simulink model "modelo_BDA"  (R2021b)
settings: Solver=ode3  StartTime=0.0  StopTime=10.0  FixedStep=1e-6  RelTol=1e-3
(part 3 of 4)

== matlab function modelo_BDA/g ==
  data: q1 input; g output; q2 input; q3 input; q4 input; q5 input; q6 input
function g = g(q1,q2,q3,q4,q5,q6)
%#codegen

%    This function was generated by the Symbolic Math Toolbox version 9.0.
%    01-Dec-2021 19:55:37

t2 = cos(q2);
t3 = cos(q4);
t4 = cos(q5);
t5 = cos(q6);
t6 = sin(q2);
t7 = sin(q4);
t8 = sin(q5);
t9 = sin(q6);
t17 = 9.007199254740992e+15;
t10 = t2.*3.235524933e+1;
t11 = t6.*3.235524933e+1;
t12 = t2.*1.0513390433e+2;
t13 = t6.*1.0513390433e+2;
t14 = t4.*5.110348748545983e-1;
t16 = t8.*5.110348748545983e-1;
t18 = t4.*t7.*8.595599785252598e-1;
t19 = t7.*t8.*8.595599785252598e-1;
t21 = (q3.*t17)./9.007199254740992e+15;
t24 = q3.*t17.*1.110223024625157e-16i;
t15 = -t13;
t20 = -t19;
t22 = cos(t21);
t23 = sin(t21);
t25 = exp(t24);
t26 = -t24;
t32 = t11+t12;
t34 = t16+t18;
t27 = 1.0./t25;
t28 = t3.*t22;
t29 = t7.*t22;
t30 = t25-1.0;
t33 = t10+t15;
t35 = t14+t20;
t36 = t22.*1.318958611e+1;
t40 = t22.*3.422984996757468e+1;
t41 = t22.*3.079131064925427e+1;
t44 = t22.*3.73890617538038e+6;
t45 = t25.*3.694216783411725e-1;
t46 = t25.*1.305783216588275e-1;
t52 = t3.*t17.*t23.*5.673626844500105e-17;
t53 = t7.*t17.*t23.*5.673626844500105e-17;
t54 = t4.*t17.*t23.*9.543032792050485e-17;
t55 = t8.*t17.*t23.*9.543032792050485e-17;
t58 = t25.*3.269483204543573;
t60 = t25.*1.334999662191606e+1;
t62 = t3.*t17.*t23.*2.556183965391409e-15;
t63 = t17.*t23.*4.869208971920574e-15;
t64 = t7.*t17.*t23.*9.827649182848514e-15;
t65 = t7.*t17.*t23.*4.958440210927941e-15;
t67 = t3.*t17.*t23.*7.425392937311983e-15;
t68 = t25.*1.091297471081935e+1;
t70 = t25.*3.784378402378023e+6;
t71 = t25.*4.456000120203464e+1;
t74 = t8.*t17.*t23.*1.275307981867505e-14;
t75 = t3.*t17.*t23.*7.696415878211547e-15;
t76 = t8.*t17.*t23.*6.931588674426758e-15;
t77 = t3.*t17.*t23.*3.509442785897641e-15;
t78 = t7.*t17.*t23.*9.400370375208377e-11;
t81 = t4.*t17.*t23.*6.72886546633755e-17;
t82 = t8.*t17.*t23.*6.72886546633755e-17;
t83 = t17.*t23.*9.790736217417458e-22;
t85 = t17.*t23.*1.646800527103812e-21;
t86 = t3.*t17.*t23.*1.041201507489731e-13;
t91 = t17.*t23.*t32.*5.673626844500105e-17;
t31 = t30.^2;
t37 = t29.*2.286892447e+1;
t38 = t28.*6.520967601e+1;
t42 = t29.*6.185536839278779e+1;
t43 = t29.*1.356524863046341e+2;
t47 = t28.*1.656853831393741e+6;
t48 = t27.*3.694216783411725e-1;
t49 = t27.*1.305783216588275e-1;
t50 = t29.*1.835160358667313e+3;
t56 = -t53;
t57 = -t54;
t59 = t27.*3.269483204543573;
t61 = t27.*1.334999662191606e+1;
t66 = -t64;
t69 = t27.*1.091297471081935e+1;
t72 = t27.*3.784378402378023e+6;
t73 = t27.*4.456000120203464e+1;
t79 = -t78;
t80 = t29+t52;
t87 = -t83;
t88 = -t86;
t92 = t17.*t23.*t33.*9.543032792050485e-17;
t39 = -t38;
t51 = -t50;
t84 = t28+t56;
t93 = -t92;
t94 = t27.*t31.*5.499266393288274;
t95 = t27.*t31.*7.936984065608979;
t96 = t8.*t80.*4.234075154e+1;
t97 = t27.*t31.*1.835560892149977e+1;
t98 = t27.*t31.*2.649229280878313e+1;
t99 = t27.*t31.*1.558899642979572e+6;
t100 = t27.*t31.*t32.*2.196325630278387e-1;
t101 = t27.*t31.*t33.*2.196325630278387e-1;
t104 = t4.*t80.*4.605359747732407e+2;
t106 = t8.*t80.*4.605359747732407e+2;
t109 = t5.*t80.*1.40259874879e-5;
t110 = t9.*t80.*1.40259874879e-5;
t113 = t45+t48+2.61156643317655e-1;
t114 = t46+t49+7.38843356682345e-1;
t89 = t4.*t84;
t90 = t8.*t84;
t102 = -t101;
t112 = -t109;
t117 = t32.*t114;
t118 = t33.*t113;
t126 = t63+t91+t93;
t129 = t58+t59+t95+1.849951749091285e+1;
t132 = t36+t60+t61+t94+9.437562846167879;
t103 = t89.*7.263507131821755e+1;
t105 = t89.*1.336375981993753e+2;
t107 = t89.*7.051076542399408e-1;
t108 = t90.*7.051076542399408e-1;
t115 = t55+t89;
t116 = t57+t90;
t119 = -t118;
t122 = t9.*(t54-t90).*(-1.40259874879e-5);
t123 = t5.*(t54-t90).*(-1.40259874879e-5);
t124 = t9.*(t54-t90).*1.40259874879e-5;
t125 = t5.*(t54-t90).*1.40259874879e-5;
t127 = t7.*t126;
t128 = t3.*t126;
t130 = t3.*t129;
t131 = t7.*t129;
t133 = t4.*t132;
t137 = t102+t117+t129;
t111 = -t108;
t120 = t5.*t115.*4.360410618e+1;
t121 = t9.*t115.*4.360410618e+1;
t134 = t37+t67+t131;
t135 = t38+t66+t130;
t138 = t3.*t137;
t139 = t7.*t137;
t141 = t100+t119+t132;
t136 = t8.*t134;
t140 = -t138;
t142 = t4.*t141;
t144 = t37+t62+t128+t139;
t143 = t96+t133+t136;
t145 = t8.*t144;
t146 = t39+t65+t127+t140;
t147 = t96+t142+t145;
et1 = t40+t71+t73+t87+t97-t118.*3.33782865+t27.*t31.*t32.*7.330958613472507e-1;
et2 = 3.150096765411469e+1;
et3 = t41+t68+t69+t85+t98+t117.*3.33782865-t27.*t31.*t33.*7.330958613472507e-1;
et4 = 6.174821949234504e+1;
et5 = t17.*t23.*2.126613508315838e-14;
et6 = t17.*t23.*t32.*1.893759423098155e-16-t17.*t23.*t33.*3.18530082611956e-16;
et7 = t44+t47+t51+t70+t72+t79+t88+t99-t118.*2.834741093616e+5-cos(q1).*4.710921170210926e+6-sin(q1).*2.435931843645872e+7;
et8 = t5.*(t76+t103+t112+t121+t124+t5.*t147.*7.26735103+t9.*(t38-t65-t127+t138).*7.26735103).*9.81e+3-t9.*(t74+t105+t110+t120+t125-t9.*t147.*7.26735103+t5.*(t38-t65-t127+t138).*7.26735103).*9.81e+3;
et9 = t8.*(t42+t77+t81+t104+t111+t4.*t144.*1.087689656e+1-t8.*t141.*1.087689656e+1).*-9.81e+3+t4.*(t43+t75+t82+t106+t107+t142.*1.087689656e+1+t145.*1.087689656e+1).*9.81e+3;
et10 = t6.*(t2.*2.143246204038348e+3+t6.*6.595899367493489e+2+3.22231575312482e+2).*-9.81e+3;
et11 = t2.*(t2.*(-6.595899367493489e+2)+t6.*2.143246204038348e+3+4.573234736449676e+2).*9.81e+3;
et12 = t113.*(et1+et2).*9.81e+3+t27.*t31.*(et3+et4).*2.154595443303097e+3+t17.*t23.*(et5+et6).*9.361715169001526e-13;
et13 = t27.*t31.*t32.*6.226014519112204e+4;
et14 = 2.675304722361566e+6;
et15 = t27.*t31.*(t41+t68+t69+t85+t98+6.174821949234504e+1);
et16 = 2.154595443303097e+3;
et17 = t2.*4.486343276457132e+6-t6.*3.161091753815448e+6+t44+t47+t51+t70+t72+t79+t88+t99;
et18 = t8.*(t42+t77+t81+t104+t111+t4.*t134.*1.087689656e+1-t8.*t132.*1.087689656e+1).*-9.81e+3+t4.*(t43+t75+t82+t106+t107+t133.*1.087689656e+1+t136.*1.087689656e+1).*9.81e+3;
et19 = t113.*(t40+t71+t73+t87+t97+3.150096765411469e+1).*9.81e+3;
et20 = t5.*(t76+t103+t112+t121+t124+t9.*t135.*7.26735103+t5.*t143.*7.26735103).*9.81e+3-t9.*(t74+t105+t110+t120+t125+t5.*t135.*7.26735103-t9.*t143.*7.26735103).*9.81e+3;
et21 = t23.^2.*1.615189683870664e+6+et15.*et16;
et22 = 2.675304722361566e+6;
et23 = t8.*3.711905458116013e+1+t3.*t5.*1.205617750389489e-5;
et24 = t4.*t7.*6.243420034246779e+1+t7.*t9.*3.583624485303893e+2;
et25 = t9.*t34.*4.360410618e+1+t9.*t35.*1.40259874879e-5;
et26 = t3.*t5.*t8.*(-3.583624485303893e+2);
et27 = t3.*5.316839912737671e+1-t4.*3.603346018435275e-1;
et28 = t3.*t4.*5.363537921262857e+2+t7.*t8.*6.060823201364798e-1;
et29 = t3.*1.166014482149094e+2-t8.*3.603346018435275e-1;
et30 = t3.*t8.*5.363537921262857e+2-t4.*t7.*6.060823201364798e-1;
et31 = t8.*6.829347327168682e+1+t4.*t7.*1.148695310384223e+2;
et32 = t3.*t9.*(-1.205617750389489e-5)+t5.*t7.*3.583624485303893e+2;
et33 = t5.*t34.*4.360410618e+1+t5.*t35.*1.40259874879e-5+t3.*t8.*t9.*3.583624485303893e+2;
et34 = t3.*1.577430398486484e+3;
et35 = t7.*1.424165243732298e+6;
et36 = t25.*5.375540669764222e-2;
et37 = t27.*5.375540669764222e-2+t5.*(et23+et24+et25+et26).*9.81e+3;
et38 = t17.*t23.*(-8.401513276977369e-12);
et39 = t27.*t31.*1.900075495889897e-2+t8.*(et27+et28).*9.81e+3-t4.*(et29+et30).*9.81e+3;
et40 = t9.*(et31+et32+et33).*-9.81e+3+3.800150991779794e-2;
et41 = t9.*(t8.*1.336375981993753e+2+t4.*t5.*1.40259874879e-5+t5.*t8.*4.360410618e+1).*-9.81e+3;
et42 = t5.*(t8.*7.263507131821755e+1+t4.*t9.*1.40259874879e-5+t8.*t9.*4.360410618e+1).*9.81e+3;
et43 = t4.*1.33075089064846e+6-t8.*6.068011639332482e+5;
et44 = t5.^2.*(-1.37594937256299e-1)-t9.^2.*1.37594937256299e-1;
g = [et7+et8+et9+et10+et11+et12+et13+et14;et17+et18+et19+et20+et21+et22;et34+et35+et36+et37+et38+et39+et40;et41+et42;et43+et44;t5.*7.125500496317142e+5-t9.*1.310984838335871e+6];

== matlab function modelo_BDA/K ==
  data: dq input; K output; q input
function K = K(dq,q)
%#codegen
dq1 = dq(1);
dq2 = dq(2);
dq3 = dq(3);
dq4 = dq(4);
dq5 = dq(5);
dq6 = dq(6);

q2 = q(2);
q3 = q(3);
q4 = q(4);
q5 = q(5);
q6 = q(6);
%    This function was generated by the Symbolic Math Toolbox version 9.0.
%    01-Dec-2021 19:55:52

t2 = cos(q2);
t3 = cos(q4);
t4 = cos(q5);
t5 = cos(q6);
t6 = sin(q2);
t7 = sin(q4);
t8 = sin(q5);
t9 = sin(q6);
t19 = 9.007199254740992e+15;
t10 = t2.*3.235524933e+1;
t11 = t6.*3.235524933e+1;
t12 = t2.*1.0513390433e+2;
t13 = t6.*1.0513390433e+2;
t14 = t4.*5.110348748545983e-1;
t16 = t8.*5.110348748545983e-1;
t17 = t5.*t8.*4.360410618e+1;
t18 = t8.*t9.*4.360410618e+1;
t20 = t3.*5.157359871151559;
t21 = t4.*t7.*8.595599785252598e-1;
t22 = t3.*t9.*8.595599785252598e-1;
t23 = t7.*t8.*8.595599785252598e-1;
t24 = t3.*t5.*8.595599785252598e-1;
t26 = (q3.*t19)./9.007199254740992e+15;
t29 = q3.*t19.*1.110223024625157e-16i;
t36 = t8.*7.263507131821755e+1;
t37 = t9.*7.263507131821755e+1;
t38 = t5.*1.336375981993753e+2;
t39 = t8.*1.336375981993753e+2;
t42 = t4.*1.356524863046341e+2;
t43 = t3.*3.748034457169395e+1;
t44 = t4.*t9.*1.336375981993753e+2;
t45 = t8.*6.185536839278779e+1;
t46 = t4.*t5.*7.263507131821755e+1;
t47 = t5.*t8.*8.018255891962515e+2;
t50 = t8.*t9.*4.358104279093053e+2;
t51 = t3.*t4.*4.931128922368695e+1;
t52 = t5.*t7.*4.931128922368695e+1;
t53 = t7.*t9.*4.931128922368695e+1;
t54 = t4.*t5.*1.40259874879e-5;
t55 = t4.*t9.*1.40259874879e-5;
t57 = t3.*t8.*t9.*4.931128922368695e+1;
t58 = t5.*t8.*8.415592492740001e-5;
t59 = t8.*t9.*8.415592492740001e-5;
t61 = t3.*t5.*t8.*4.931128922368695e+1;
t71 = t3.*9.473039288601392e+2;
t72 = t7.*9.473039288601392e+2;
t76 = t4.*7.291450524218959e+2;
t77 = t8.*7.291450524218959e+2;
t79 = t5.*1.246862890394724e+3;
t80 = t9.*1.246862890394724e+3;
t82 = t2.*1.908064859676306e+4;
t83 = t8.*6.829347327168682e+1;
t85 = t8.*3.711905458116013e+1;
t86 = t3.*6.892171862305337e+2;
t87 = t8.*4.200920957332826e+3;
t89 = t6.*5.850608528728732e+4;
t90 = t3.*3.746052020548068e+2;
t91 = t3.*5.316839912737671e+1;
t94 = t4.*6.932315136240378e+1;
t95 = t8.*3.161025044569338e+1;
t97 = t4.*t7.*6.243420034246779e+1;
t98 = t3.*t9.*6.243420034246779e+1;
t99 = t5.*t7.*3.583624485303893e+2;
t100 = t7.*t9.*3.583624485303893e+2;
t101 = t4.*2.524704765397172;
t102 = t4.*t5.*(-1.246862890394724e+3);
t103 = t7.*1.451748464558917e+2;
t104 = t4.*t9.*(-1.246862890394724e+3);
t105 = t3.*1.166014482149094e+2;
t106 = t3.*t5.*1.148695310384223e+2;
t107 = t4.*t7.*1.148695310384223e+2;
t109 = t3.*t4.*3.583624485303893e+2;
t110 = t8.*3.603346018435275e-1;
t111 = t4.*t7.*5.316839912737671e+1;
t112 = t7.*5.363537921262857e+2;
t113 = t8.*1.758766552463174e+1;
t114 = t4.*3.603346018435275e-1;
t116 = t5.*3.146556876441599e-4;
t117 = t8.*3.146556876441599e-4;
t118 = t7.*t8.*1.166014482149094e+2;
t119 = t3.*t5.*t8.*3.583624485303893e+2;
t120 = t8.*4.126305645247942e-4;
t121 = t9.*4.126305645247942e-4;
t122 = t3.*t8.*t9.*3.583624485303893e+2;
t124 = t3.*1.607982057580514e-1;
t125 = t3.*t4.*5.363537921262857e+2;
t126 = t3.*t8.*5.363537921262857e+2;
t129 = t4.*t7.*6.060823201364798e-1;
t130 = t4.*t9.*3.146556876441599e-4;
t131 = t7.*t8.*6.060823201364798e-1;
t132 = t4.*t5.*4.126305645247942e-4;
t134 = t3.*t5.*1.205617750389489e-5;
t135 = t3.*t9.*1.205617750389489e-5;
t137 = t8.*5.878411097842592e+2;
t139 = t4.*2.257319383180457e+3;
t143 = t5.*3.383303336574349e+3;
t144 = t9.*1.744166601788531e+3;
t146 = t4.*t5.*1.744166601788531e+3;
t147 = t4.*t9.*3.383303336574349e+3;
t155 = t3.*2.748657914322168e+3;
t163 = t4.*3.726185506152731e+2;
t164 = t8.*3.726185506152731e+2;
t165 = t3.*2.286243086622337e+3;
t166 = t8.*2.14681711570464e+3;
t167 = t7.*6.685860485757689;
t170 = t7.*3.050167960854463e+3;
t171 = t7.*6.689198986080043e+3;
t175 = t3.*t4.*3.581729009555754e+3;
t176 = t7.*t9.*3.581729009555754e+3;
t177 = t4.*t7.*3.610943527871318e+3;
t178 = t4.*t7.*6.267439056015643e+2;
t179 = t3.*t5.*1.071753439291633e+3;
t180 = t7.*t8.*6.267439056015643e+2;
t181 = t3.*t9.*1.071753439291633e+3;
t182 = t3.*t4.*6.589842255968259e+3;
t185 = t5.*t7.*6.589842255968259e+3;
t186 = t7.*3.119613856461354e+4;
t187 = t3.*t4.*3.050167960854463e+3;
t189 = t3.*2.170135173927414;
t191 = t3.*t8.*6.689198986080043e+3;
t192 = t8.*2.108686089031105e-4;
t193 = t8.*8.987910450364716;
t194 = t4.*1.290212183829552;
t195 = t3.*1.511765340066191e+1;
t196 = t3.*t8.*t9.*6.589842255968259e+3;
t199 = t3.*t5.*t8.*3.581729009555754e+3;
t201 = t8.*1.608000299575208e-4;
t202 = t7.*t8.*2.170135173927414;
t203 = t3.*1.454828146091616;
t204 = t7.*1.454828146091616;
t206 = t3.*t4.*3.476976747206118e+1;
t207 = t3.*t8.*3.476976747206118e+1;
t208 = t4.*t7.*1.511765340066191e+1;
t210 = t4.*t7.*3.54680719181798e-4;
t211 = t3.*t9.*3.54680719181798e-4;
t213 = t3.*t5.*2.704654361142649e-4;
t214 = t5.*t7.*6.916395256636513e-4;
t215 = t4.*t7.*2.704654361142649e-4;
t216 = t7.*t9.*6.916395256636513e-4;
t220 = t8.*3.004073079729871e+2;
t221 = t3.*t5.*t8.*6.916395256636513e-4;
t222 = t3.*t8.*t9.*6.916395256636513e-4;
t224 = t4.*1.153568928490484e+3;
t226 = t7.*t8.*1.940301400531246e+3;
t227 = t4.*t7.*5.052846917024227e+2;
t232 = t3.*2.862617746347316e+4;
t246 = t3.*t5.*2.908152143330287e+3;
t247 = t3.*t9.*1.499215806777825e+3;
t15 = -t13;
t25 = -t23;
t27 = cos(t26);
t28 = sin(t26);
t30 = exp(t29);
t31 = -t29;
t48 = -t44;
t49 = -t45;
t56 = t11+t12;
t62 = -t61;
t63 = t16+t21;
t84 = -t77;
t92 = t4.*t79;
t93 = t4.*t80;
t96 = -t90;
t108 = -t94;
t115 = -t110;
t123 = -t114;
t127 = -t119;
t128 = -t121;
t133 = -t129;
t136 = -t135;
t138 = -t137;
t140 = t20+t51;
t160 = -t155;
t168 = -t163;
t188 = -t175;
t190 = -t179;
t197 = -t193;
t198 = -t194;
t200 = -t195;
t205 = -t199;
t212 = -t207;
t218 = -t208;
t219 = -t211;
t223 = -t221;
t225 = -t224;
t250 = -t247;
t272 = t37+t38+4.360410618e+1;
t277 = t18+t36+t55;
t279 = t17+t39+t54;
t300 = t71-8.631091645042425e+1;
t301 = t72+9.559948463095517e-2;
t308 = t101+t113;
t309 = t103+t124;
t438 = t79+t144+4.358104279093053e+2;
t441 = t80+t143+8.018255891962515e+2;
t524 = t186+t203+2.538346896821816;
t525 = t58+t104+t120+t146;
t526 = t59+t102+t117+t147;
t530 = t204+t232-3.371409213983255e+2;
t549 = t47+t50+t87+t130+t132;
t32 = 1.0./t30;
t33 = t3.*t27;
t34 = t7.*t27;
t40 = t30-1.0;
t60 = t10+t15;
t64 = t14+t25;
t66 = t5.*t63.*6.0;
t68 = t9.*t63.*6.0;
t70 = t27.*1.318958611e+1;
t141 = t5.*t63.*4.360410618e+1;
t142 = t9.*t63.*4.360410618e+1;
t149 = t27.*3.811321279694577e+2;
t150 = t27.*3.422984996757468e+1;
t154 = t27.*3.079131064925427e+1;
t169 = t30.*3.694216783411725e-1;
t172 = t30.*1.305783216588275e-1;
t209 = t42+t49;
t217 = t46+t48;
t229 = t9.*t63.*4.358104279093053e+2;
t231 = t5.*t63.*8.018255891962515e+2;
t234 = t5.*t63.*8.415592492740001e-5;
t235 = t9.*t63.*8.415592492740001e-5;
t238 = t3.*t19.*t28.*5.673626844500105e-17;
t239 = t7.*t19.*t28.*5.673626844500105e-17;
t240 = t4.*t19.*t28.*9.543032792050485e-17;
t241 = t8.*t19.*t28.*9.543032792050485e-17;
t242 = t3.*t19.*t28.*3.404176106700063e-16;
t245 = t27.*2.227646919556693e+3;
t249 = t27.*8.579529175625027e+2;
t253 = t27.*2.467380792691235;
t256 = t30.*3.269483204543573;
t261 = t30.*1.334999662191606e+1;
t268 = t27.*1.104616756676389e-4;
t269 = t27.*5.202289239433555e-4;
t282 = t3.*t19.*t28.*2.556183965391409e-15;
t283 = t7.*t19.*t28.*2.556183965391409e-15;
t284 = t19.*t28.*4.869208971920574e-15;
t285 = t7.*t19.*t28.*9.827649182848514e-15;
t286 = t3.*t19.*t28.*2.473934273532809e-15;
t289 = t7.*t19.*t28.*4.958440210927941e-15;
t290 = t7.*t19.*t28.*7.425392937311983e-15;
t292 = t3.*t19.*t28.*7.425392937311983e-15;
t294 = t30.*3.857674212413887e+2;
t296 = t30.*1.091297471081935e+1;
t302 = t30.*4.456000120203464e+1;
t303 = t27.*3.608035586078749e-4;
t310 = t116+t128;
t311 = t76+t138;
t312 = t84+t139;
t313 = t8.*t19.*t28.*1.275307981867505e-14;
t314 = t3.*t19.*t28.*4.549259187470966e-14;
t315 = t19.*t28.*1.611764571317528e-14;
t316 = t3.*t19.*t28.*1.117556177536684e-13;
t317 = t7.*t19.*t28.*1.117556177536684e-13;
t319 = t3.*t19.*t28.*2.524584390187751e-13;
t320 = t7.*t19.*t28.*2.524584390187751e-13;
t321 = t7.*t19.*t28.*1.068943235898118e-13;
t322 = t3.*t19.*t28.*7.696415878211547e-15;
t323 = t7.*t19.*t28.*5.39324412732078e-14;
t324 = t4.*t19.*t28.*1.294536125128302e-14;
t326 = t7.*t19.*t28.*9.582436671975919e-15;
t327 = t8.*t19.*t28.*6.931588674426758e-15;
t328 = t3.*t19.*t28.*2.472625742899312e-14;
t331 = t19.*t28.*1.78521870351002e-17;
t334 = t3.*t19.*t28.*3.509442785897641e-15;
t336 = t8.*t19.*t28.*5.90287808936737e-15;
t337 = t3.*t19.*t28.*1.061367489795852e-17;
t338 = t19.*t28.*2.126613508315838e-14;
t341 = t4.*t19.*t28.*6.72886546633755e-17;
t342 = t8.*t19.*t28.*6.72886546633755e-17;
t343 = t19.*t28.*9.790736217417458e-22;
t345 = t19.*t28.*1.646800527103812e-21;
t352 = t30.*2.254739352916933e+3;
t353 = t19.*t28.*t56.*5.673626844500105e-17;
t356 = t30.*2.497388846980927;
t358 = t30.*5.576400544494359e+2;
t361 = t30.*5.642007925493603e-5;
t367 = t30.*2.303752062145191e-4;
t369 = t19.*t28.*6.295748150968656e-14;
t370 = t7.*t19.*t28.*3.067061459005602e-13;
t371 = t7.*t19.*t28.*6.726247428052494e-13;
t372 = t7.*t19.*t28.*6.078928606401748e-13;
t374 = t7.*t19.*t28.*1.333145046183106e-12;
t376 = t4.*t19.*t28.*6.958255145423523e-14;
t377 = t8.*t19.*t28.*4.008952645263927e-13;
t378 = t8.*t19.*t28.*6.958255145423523e-14;
t380 = t3.*t19.*t28.*1.509061667990639e-13;
t381 = t3.*t19.*t28.*1.657497724402608e-13;
t385 = t3.*t19.*t28.*4.691552578623493e-13;
t386 = t3.*t19.*t28.*1.291537270195008e-12;
t387 = t19.*t28.*4.740092871521216e-16;
t388 = t8.*t19.*t28.*1.678396688371765e-15;
t389 = t3.*t19.*t28.*1.432423273139473e-16;
t390 = t3.*t19.*t28.*9.978585125263967e-16;
t391 = t4.*t19.*t28.*2.409334036643134e-16;
t392 = t7.*t19.*t28.*7.599994046755678e-16;
t394 = t3.*t19.*t28.*9.602764472540121e-17;
t395 = t8.*t19.*t28.*3.002769545393412e-20;
t396 = t7.*t19.*t28.*9.602764472540121e-17;
t397 = t7.*t19.*t28.*6.448744418276857e-12;
t398 = t7.*t19.*t28.*3.19687103847679e-12;
t399 = t19.*t28.*4.337843352208199e-20;
t406 = t7.*t19.*t28.*1.670884143038041e-15;
t407 = t8.*t19.*t28.*3.937747008262415e-20;
t412 = t8.*t19.*t28.*5.609786987186535e-14;
t413 = t19.*t28.*3.910962660750154e-13;
t414 = t4.*t19.*t28.*2.154167289582227e-13;
t415 = t19.*t28.*t56.*1.893759423098155e-16;
t419 = t3.*t19.*t28.*3.027237730074418e-12;
t421 = t3.*t19.*t28.*6.279111109874485e-12;
t426 = t30.*2.268539354478371e-4;
t428 = t19.*t28.*2.007862416620223e-13;
t429 = t19.*t28.*2.261065882456945e-13;
t434 = t19.*t28.*5.703946554323684e-14;
t447 = t19.*t28.*t56.*1.74698406676951e-15;
t449 = t19.*t28.*t56.*1.942073956592427e-15;
t454 = t19.*t28.*1.428243658465093e-13;
t486 = t19.*t28.*t56.*5.091700655507849e-16;
t523 = t160+t167+2.094342917444822e+3;
t533 = t91+t123+t125+t131;
t534 = t105+t115+t126+t133;
t578 = t95+t108+t111+t112+t118;
t656 = t165+t187+t191+t197+t198+t202+t218;
t657 = t164+t171+t178+t189+t206+t225+t226;
t658 = t168+t170+t180+t200+t212+t220+t227;
t35 = t34.*6.0;
t41 = t40.^2;
t65 = t5.*t64;
t67 = t9.*t64;
t73 = t34.*4.360410618e+1;
t74 = t33.*2.286892447e+1;
t75 = t34.*2.286892447e+1;
t81 = t33.*6.520967601e+1;
t151 = t34.*4.358104279093053e+2;
t152 = t33.*1.328674864713371e+3;
t153 = t34.*1.328674864713371e+3;
t156 = t34.*8.018255891962515e+2;
t157 = t34.*6.185536839278779e+1;
t158 = t33.*1.688943762888624e+2;
t159 = t34.*1.356524863046341e+2;
t162 = t33.*7.092789006718835e+2;
t173 = t34.*1.870703729528352e-1;
t174 = t32.*3.694216783411725e-1;
t183 = t32.*1.305783216588275e-1;
t243 = -t239;
t244 = -t240;
t248 = t34.*4.522154679359383e+3;
t251 = t34.*2.65978307941329e+3;
t252 = t34.*2.92140771649329e+3;
t254 = t33.*4.033568532372886e+3;
t255 = t33.*8.84585468187615e+3;
t258 = t33.*9.245169992678717;
t259 = t32.*3.269483204543573;
t260 = t34.*2.524704765397172;
t263 = t33.*4.153012702745543e+4;
t264 = t34.*1.758766552463174e+1;
t265 = t32.*1.334999662191606e+1;
t266 = t33.*1.692526621106363;
t267 = t34.*1.692526621106363;
t271 = -t268;
t273 = -t269;
t274 = t34.*3.854027039691565e+4;
t291 = -t285;
t293 = -t290;
t295 = t34.*2.310978750639558e+3;
t297 = t32.*3.857674212413887e+2;
t298 = t32.*1.091297471081935e+1;
t299 = t33.*4.724604290218056;
t304 = t32.*4.456000120203464e+1;
t305 = -t303;
t318 = -t314;
t325 = -t317;
t329 = -t320;
t330 = -t321;
t332 = -t323;
t333 = -t324;
t335 = -t326;
t339 = -t337;
t340 = t34+t238;
t346 = -t343;
t354 = t32.*2.254739352916933e+3;
t355 = t19.*t28.*t60.*9.543032792050485e-17;
t359 = t32.*2.497388846980927;
t360 = t32.*5.576400544494359e+2;
t362 = t32.*5.642007925493603e-5;
t364 = t52+t57+t66;
t365 = t53+t62+t68;
t368 = t32.*2.303752062145191e-4;
t373 = -t369;
t375 = -t370;
t379 = -t372;
t382 = -t374;
t383 = -t376;
t384 = -t378;
t393 = -t389;
t400 = -t392;
t401 = -t394;
t402 = -t395;
t403 = -t396;
t404 = -t397;
t405 = -t398;
t408 = -t399;
t409 = -t406;
t416 = -t414;
t417 = t19.*t28.*t60.*3.18530082611956e-16;
t420 = -t419;
t423 = -t421;
t427 = t32.*2.268539354478371e-4;
t430 = -t428;
t450 = -t447;
t452 = t19.*t28.*t60.*2.938424872360468e-15;
t456 = t19.*t28.*t60.*3.266565807075334e-15;
t491 = t19.*t28.*t60.*8.564233717611997e-16;
t581 = t19.*t28.*t523.*9.543032792050485e-17;
t69 = -t65;
t78 = -t74;
t88 = -t81;
t145 = t24+t67;
t161 = -t156;
t184 = -t173;
t228 = t67.*1.336375981993753e+2;
t230 = t65.*7.263507131821755e+1;
t236 = t65.*1.40259874879e-5;
t237 = t67.*1.40259874879e-5;
t257 = -t255;
t262 = -t260;
t270 = -t267;
t275 = -t274;
t276 = t65.*1.246862890394724e+3;
t278 = t67.*1.246862890394724e+3;
t287 = t65.*4.126305645247942e-4;
t288 = t67.*3.146556876441599e-4;
t306 = t65.*1.744166601788531e+3;
t307 = t67.*3.383303336574349e+3;
t344 = t33+t243;
t347 = t5.*t340;
t348 = t9.*t340;
t357 = -t355;
t363 = t32.*t41.*5.499266393288274;
t366 = t32.*t41.*7.936984065608979;
t410 = t4.*t340.*4.234075154e+1;
t411 = t8.*t340.*4.234075154e+1;
t418 = -t417;
t422 = t32.*t41.*1.589092398552061e+2;
t424 = t32.*t41.*1.835560892149977e+1;
t425 = t32.*t41.*2.649229280878313e+1;
t431 = t32.*t41.*t56.*2.196325630278387e-1;
t432 = t32.*t41.*t60.*2.196325630278387e-1;
t435 = t4.*t340.*3.077051043151931e+2;
t436 = t37.*t340;
t437 = t38.*t340;
t443 = t4.*t340.*4.605359747732407e+2;
t445 = t8.*t340.*4.605359747732407e+2;
t460 = -t456;
t461 = t32.*t41.*9.287951675407251e+2;
t462 = t32.*t41.*1.02874981515943;
t463 = t32.*t41.*4.326292055563303e+2;
t464 = t32.*t41.*1.369651538214088e-4;
t465 = t32.*t41.*9.489849812415379e-5;
t466 = t32.*t41.*t56.*6.34659991754557;
t467 = t32.*t41.*t56.*7.330958613472507e-1;
t468 = t32.*t41.*t60.*7.330958613472507e-1;
t470 = t4.*t340.*5.658316341762099e+3;
t471 = t4.*t340.*3.07542350777483e+3;
t472 = t4.*t340.*2.619002784534197e+3;
t473 = t4.*t340.*4.465233410425356e+3;
t474 = t8.*t340.*5.743628218407764e+3;
t475 = t79.*t340;
t477 = t80.*t340;
t481 = t4.*t340.*2.985478799712556e+1;
t482 = t8.*t340.*2.985478799712556e+1;
t488 = t121.*t340;
t489 = t116.*t340;
t500 = t169+t174+2.61156643317655e-1;
t501 = t172+t183+7.38843356682345e-1;
t502 = t32.*t41.*1.515649212522415e-4;
t503 = t32.*t41.*t56.*3.709470474531108e+1;
t504 = t32.*t41.*t56.*7.517989680436807;
t505 = t32.*t41.*t56.*4.108674547820486e-2;
t506 = t32.*t41.*t60.*6.762774476882097;
t508 = t143.*t340;
t509 = t144.*t340;
t510 = t32.*t41.*t56.*3.790105603165286e-6;
t512 = t32.*t41.*t60.*3.790105603165286e-6;
t514 = t32.*t41.*t56.*3.25782309086522e-6;
t515 = t32.*t41.*t60.*1.936876142599284e-6;
t535 = t308.*t340;
t591 = t340.*t530;
t682 = t340.*t656;
t148 = t22+t69;
t233 = -t230;
t280 = -t276;
t281 = -t278;
t349 = t4.*t344;
t350 = t8.*t344;
t351 = -t348;
t433 = -t432;
t439 = t348.*4.358104279093053e+2;
t442 = t347.*8.018255891962515e+2;
t455 = t347.*1.40259874879e-5;
K = ft_1({dq1,dq2,dq3,dq4,dq5,dq6,t100,t106,t107,t109,t122,t127,t134,t136,t140,t141,t142,t145,t148,t149,t150,t151,t152,t153,t154,t156,t157,t158,t159,t161,t162,t166,t176,t177,t181,t182,t184,t185,t188,t19,t190,t191,t192,t196,t197,t198,t2,t201,t202,t205,t209,t210,t213,t214,t215,t216,t218,t219,t222,t223,t228,t229,t231,t233,t234,t235,t236,t237,t240,t241,t242,t244,t245,t246,t248,t249,t250,t251,t252,t253,t254,t255,t256,t257,t258,t259,t260,t261,t262,t263,t264,t265,t266,t27,t270,t271,t272,t273,t275,t277,t279,t28,t280,t281,t282,t283,t284,t286,t287,t288,t289,t291,t292,t293,t294,t295,t296,t297,t298,t299,t3,t300,t301,t302,t304,t305,t306,t307,t308,t309,t310,t311,t312,t313,t314,t315,t316,t318,t319,t322,t325,t327,t328,t329,t330,t331,t332,t333,t334,t335,t336,t338,t339,t340,t341,t342,t344,t345,t346,t347,t348,t349,t35,t350,t351,t352,t353,t354,t356,t357,t358,t359,t36,t360,t361,t362,t363,t364,t365,t366,t367,t368,t37,t371,t373,t374,t375,t377,t378,t379,t38,t380,t381,t382,t383,t384,t385,t386,t387,t388,t389,t39,t390,t391,t393,t395,t4,t400,t401,t402,t403,t404,t405,t407,t408,t409,t410,t411,t412,t413,t414,t415,t416,t418,t42,t420,t422,t423,t424,t425,t426,t427,t429,t43,t430,t431,t433,t434,t435,t436,t437,t438,t439,t44,t441,t442,t443,t445,t449,t45,t450,t452,t454,t455,t46,t460,t461,t462,t463,t464,t465,t466,t467,t468,t470,t471,t472,t473,t474,t475,t477,t481,t482,t486,t488,t491,t5,t500,t501,t502,t503,t504,t505,t506,t508,t509,t51,t510,t512,t514,t515,t523,t524,t525,t526,t530,t533,t534,t535,t549,t56,t578,t581,t591,t6,t60,t63,t64,t65,t656,t657,t658,t67,t682,t7,t70,t73,t74,t75,t76,t77,t78,t79,t8,t80,t81,t82,t83,t85,t86,t88,t89,t9,t90,t96,t97,t98,t99});
end
function K = ft_1(ct)
dq1 = ct{1};
dq2 = ct{2};
dq3 = ct{3};
dq4 = ct{4};
dq5 = ct{5};
dq6 = ct{6};
t100 = ct{7};
t106 = ct{8};
t107 = ct{9};
t109 = ct{10};
t122 = ct{11};
t127 = ct{12};
t134 = ct{13};
t136 = ct{14};
t140 = ct{15};
t141 = ct{16};
t142 = ct{17};
t145 = ct{18};
t148 = ct{19};
t149 = ct{20};
t150 = ct{21};
t151 = ct{22};
t152 = ct{23};
t153 = ct{24};
t154 = ct{25};
t156 = ct{26};
t157 = ct{27};
t158 = ct{28};
t159 = ct{29};
t161 = ct{30};
t162 = ct{31};
t166 = ct{32};
t176 = ct{33};
t177 = ct{34};
t181 = ct{35};
t182 = ct{36};
t184 = ct{37};
t185 = ct{38};
t188 = ct{39};
t19 = ct{40};
t190 = ct{41};
t191 = ct{42};
t192 = ct{43};
t196 = ct{44};
t197 = ct{45};
t198 = ct{46};
t2 = ct{47};
t201 = ct{48};
t202 = ct{49};
t205 = ct{50};
t209 = ct{51};
t210 = ct{52};
t213 = ct{53};
t214 = ct{54};
t215 = ct{55};
t216 = ct{56};
t218 = ct{57};
t219 = ct{58};
t222 = ct{59};
t223 = ct{60};
t228 = ct{61};
t229 = ct{62};
t231 = ct{63};
t233 = ct{64};
t234 = ct{65};
t235 = ct{66};
t236 = ct{67};
t237 = ct{68};
t240 = ct{69};
t241 = ct{70};
t242 = ct{71};
t244 = ct{72};
t245 = ct{73};
t246 = ct{74};
t248 = ct{75};
t249 = ct{76};
t250 = ct{77};
t251 = ct{78};
t252 = ct{79};
t253 = ct{80};
t254 = ct{81};
t255 = ct{82};
t256 = ct{83};
t257 = ct{84};
t258 = ct{85};
t259 = ct{86};
t260 = ct{87};
t261 = ct{88};
t262 = ct{89};
t263 = ct{90};
t264 = ct{91};
t265 = ct{92};
t266 = ct{93};
t27 = ct{94};
t270 = ct{95};
t271 = ct{96};
t272 = ct{97};
t273 = ct{98};
t275 = ct{99};
t277 = ct{100};
t279 = ct{101};
t28 = ct{102};
t280 = ct{103};
t281 = ct{104};
t282 = ct{105};
t283 = ct{106};
t284 = ct{107};
t286 = ct{108};
t287 = ct{109};
t288 = ct{110};
t289 = ct{111};
t291 = ct{112};
t292 = ct{113};
t293 = ct{114};
t294 = ct{115};
t295 = ct{116};
t296 = ct{117};
t297 = ct{118};
t298 = ct{119};
t299 = ct{120};
t3 = ct{121};
t300 = ct{122};
t301 = ct{123};
t302 = ct{124};
t304 = ct{125};
t305 = ct{126};
t306 = ct{127};
t307 = ct{128};
t308 = ct{129};
t309 = ct{130};
t310 = ct{131};
t311 = ct{132};
t312 = ct{133};
t313 = ct{134};
t314 = ct{135};
t315 = ct{136};
t316 = ct{137};
t318 = ct{138};
t319 = ct{139};
t322 = ct{140};
t325 = ct{141};
t327 = ct{142};
t328 = ct{143};
t329 = ct{144};
t330 = ct{145};
t331 = ct{146};
t332 = ct{147};
t333 = ct{148};
t334 = ct{149};
t335 = ct{150};
t336 = ct{151};
t338 = ct{152};
t339 = ct{153};
t340 = ct{154};
t341 = ct{155};
t342 = ct{156};
t344 = ct{157};
t345 = ct{158};
t346 = ct{159};
t347 = ct{160};
t348 = ct{161};
t349 = ct{162};
t35 = ct{163};
t350 = ct{164};
t351 = ct{165};
t352 = ct{166};
t353 = ct{167};
t354 = ct{168};
t356 = ct{169};
t357 = ct{170};
t358 = ct{171};
t359 = ct{172};
t36 = ct{173};
t360 = ct{174};
t361 = ct{175};
t362 = ct{176};
t363 = ct{177};
t364 = ct{178};
t365 = ct{179};
t366 = ct{180};
t367 = ct{181};
t368 = ct{182};
t37 = ct{183};
t371 = ct{184};
t373 = ct{185};
t374 = ct{186};
t375 = ct{187};
t377 = ct{188};
t378 = ct{189};
t379 = ct{190};
t38 = ct{191};
t380 = ct{192};
t381 = ct{193};
t382 = ct{194};
t383 = ct{195};
t384 = ct{196};
t385 = ct{197};
t386 = ct{198};
t387 = ct{199};
t388 = ct{200};
t389 = ct{201};
t39 = ct{202};
t390 = ct{203};
t391 = ct{204};
t393 = ct{205};
t395 = ct{206};
t4 = ct{207};
t400 = ct{208};
t401 = ct{209};
t402 = ct{210};
t403 = ct{211};
t404 = ct{212};
t405 = ct{213};
t407 = ct{214};
t408 = ct{215};
t409 = ct{216};
t410 = ct{217};
t411 = ct{218};
t412 = ct{219};
t413 = ct{220};
t414 = ct{221};
t415 = ct{222};
t416 = ct{223};
t418 = ct{224};
t42 = ct{225};
t420 = ct{226};
t422 = ct{227};
t423 = ct{228};
t424 = ct{229};
t425 = ct{230};
t426 = ct{231};
t427 = ct{232};
t429 = ct{233};
t43 = ct{234};
t430 = ct{235};
t431 = ct{236};
t433 = ct{237};
t434 = ct{238};
t435 = ct{239};
t436 = ct{240};
t437 = ct{241};
t438 = ct{242};
t439 = ct{243};
t44 = ct{244};
t441 = ct{245};
t442 = ct{246};
t443 = ct{247};
t445 = ct{248};
t449 = ct{249};
t45 = ct{250};
t450 = ct{251};
t452 = ct{252};
t454 = ct{253};
t455 = ct{254};
t46 = ct{255};
t460 = ct{256};
t461 = ct{257};
t462 = ct{258};
t463 = ct{259};
t464 = ct{260};
t465 = ct{261};
t466 = ct{262};
t467 = ct{263};
t468 = ct{264};
t470 = ct{265};
t471 = ct{266};
t472 = ct{267};
t473 = ct{268};
t474 = ct{269};
t475 = ct{270};
t477 = ct{271};
t481 = ct{272};
t482 = ct{273};
t486 = ct{274};
t488 = ct{275};
t491 = ct{276};
t5 = ct{277};
t500 = ct{278};
t501 = ct{279};
t502 = ct{280};
t503 = ct{281};
t504 = ct{282};
t505 = ct{283};
t506 = ct{284};
t508 = ct{285};
t509 = ct{286};
t51 = ct{287};
t510 = ct{288};
t512 = ct{289};
t514 = ct{290};
t515 = ct{291};
t523 = ct{292};
t524 = ct{293};
t525 = ct{294};
t526 = ct{295};
t530 = ct{296};
t533 = ct{297};
t534 = ct{298};
t535 = ct{299};
t549 = ct{300};
t56 = ct{301};
t578 = ct{302};
t581 = ct{303};
t591 = ct{304};
t6 = ct{305};
t60 = ct{306};
t63 = ct{307};
t64 = ct{308};
t65 = ct{309};
t656 = ct{310};
t657 = ct{311};
t658 = ct{312};
t67 = ct{313};
t682 = ct{314};
t7 = ct{315};
t70 = ct{316};
t73 = ct{317};
t74 = ct{318};
t75 = ct{319};
t76 = ct{320};
t77 = ct{321};
t78 = ct{322};
t79 = ct{323};
t8 = ct{324};
t80 = ct{325};
t81 = ct{326};
t82 = ct{327};
t83 = ct{328};
t85 = ct{329};
t86 = ct{330};
t88 = ct{331};
t89 = ct{332};
t9 = ct{333};
t90 = ct{334};
t96 = ct{335};
t97 = ct{336};
t98 = ct{337};
t99 = ct{338};
t457 = t348.*1.40259874879e-5;
t469 = -t468;
t476 = -t470;
t478 = t76.*t344;
t479 = t77.*t344;
t480 = t348.*(-1.246862890394724e+3);
t485 = -t481;
t495 = t347.*(-3.146556876441599e-4);
t507 = -t506;
t511 = t347.*(-3.383303336574349e+3);
t513 = -t512;
t527 = t56.*t501;
t528 = t60.*t500;
t590 = t344.*t524;
t592 = t284+t353+t357;
t595 = t256+t259+t366+1.849951749091285e+1;
t598 = t261+t265+t363+9.437562846167879;
t625 = t338+t415+t418;
t630 = t85+t97+t100+t127+t134+t142+t237;
t631 = t83+t99+t107+t122+t136+t141+t236;
t680 = t154+t296+t298+t345+t425+6.174821949234504e+1;
t681 = t150+t302+t304+t346+t424+3.150096765411469e+1;
t685 = t249+t358+t360+t408+t463+8.92670750207894e+2;
t693 = t273+t361+t362+t429+t464+3.192382947754238e-4;
t694 = t271+t367+t368+t430+t465+1.628600027717729e-4;
t729 = t149+t158+t184+t294+t297+t335+t339+t422+2.727120002407305e+2;
t732 = t166+t176+t177+t185+t196+t205+t213+t219+t229+t231+t287+t288;
t440 = t349.*7.263507131821755e+1;
t444 = t349.*1.336375981993753e+2;
t446 = t350.*1.356524863046341e+2;
t448 = t349.*6.185536839278779e+1;
t451 = t349.*7.051076542399408e-1;
t453 = t350.*7.051076542399408e-1;
t459 = -t455;
t483 = t349.*(-7.291450524218959e+2);
t484 = t349.*4.200920957332826e+3;
t487 = t350.*2.524704765397172;
t492 = t349.*1.758766552463174e+1;
t493 = t349.*4.126305645247942e-4;
t494 = t349.*3.146556876441599e-4;
t497 = t349.*5.878411097842592e+2;
t498 = t350.*2.257319383180457e+3;
t516 = t241+t349;
t517 = t244+t350;
t518 = -t5.*(t240-t350);
t520 = -t9.*(t240-t350);
t529 = -t528;
t536 = t527.*3.33782865;
t537 = t528.*2.889644336e+1;
t538 = t528.*3.33782865;
t541 = t5.*(t240-t350).*(-7.263507131821755e+1);
t544 = t9.*(t240-t350).*(-1.336375981993753e+2);
t545 = t5.*(t240-t350).*(-4.358104279093053e+2);
t546 = t5.*(t240-t350).*7.263507131821755e+1;
t547 = t9.*(t240-t350).*(-8.018255891962515e+2);
t548 = t5.*(t240-t350).*4.358104279093053e+2;
t550 = t9.*(t240-t350).*(-1.40259874879e-5);
t553 = t5.*(t240-t350).*(-1.40259874879e-5);
t554 = t9.*(t240-t350).*1.40259874879e-5;
t556 = t5.*(t240-t350).*1.40259874879e-5;
t557 = t528.*1.688943762888624e+2;
t558 = t527.*3.079131064925427e+1;
t560 = t528.*3.422984996757468e+1;
t562 = -t79.*(t240-t350);
t563 = -t80.*(t240-t350);
t564 = t528.*1.870703729528352e-1;
t565 = t5.*(t240-t350).*1.246862890394724e+3;
t567 = t527.*1.72565741205e-5;
t568 = t528.*1.72565741205e-5;
t570 = t5.*(t240-t350).*(-4.126305645247942e-4);
t571 = t9.*(t240-t350).*(-3.146556876441599e-4);
t572 = t5.*(t240-t350).*4.126305645247942e-4;
t573 = t9.*(t240-t350).*3.146556876441599e-4;
t574 = t5.*(t240-t350).*(-1.744166601788531e+3);
t575 = t9.*(t240-t350).*(-3.383303336574349e+3);
t576 = t5.*(t240-t350).*1.744166601788531e+3;
t577 = t9.*(t240-t350).*3.383303336574349e+3;
t579 = t527.*8.818711196088817e-6;
t580 = t528.*1.483306048043653e-5;
t586 = -t312.*(t240-t350);
t587 = t312.*(t240-t350);
t593 = t7.*t592;
t594 = t3.*t592;
t596 = t3.*t595;
t597 = t7.*t595;
t599 = t43+t98+t106+t109+t228+t233;
t626 = t70+t598;
t647 = -t438.*(t348+t5.*(t240-t350));
t648 = t438.*(t348+t5.*(t240-t350));
t677 = -t525.*(t348+t5.*(t240-t350));
t679 = t525.*(t348+t5.*(t240-t350));
t686 = -t657.*(t240-t350);
t688 = t433+t527+t595;
t698 = t27.*t685;
t726 = t19.*t28.*t693.*9.543032792050485e-17;
t727 = t19.*t28.*t694.*5.673626844500105e-17;
t730 = t86+t181+t182+t201+t215+t216+t223+t235+t246+t280+t307;
t731 = t96+t188+t190+t192+t210+t214+t222+t234+t250+t281+t306;
t458 = -t453;
t490 = -t487;
t496 = -t494;
t499 = -t498;
t519 = t5.*t516.*6.0;
t521 = t9.*t516.*6.0;
t531 = t5.*t516.*4.360410618e+1;
t532 = t9.*t516.*4.360410618e+1;
t539 = -t537;
t540 = t9.*t516.*4.358104279093053e+2;
t542 = -t538;
t543 = t5.*t516.*8.018255891962515e+2;
t551 = t5.*t516.*8.415592492740001e-5;
t552 = t9.*t516.*8.415592492740001e-5;
t559 = -t557;
t561 = -t560;
t566 = -t564;
t569 = -t568;
t582 = t310.*t516;
t583 = t311.*t516;
t588 = t347+t520;
t589 = t351+t518;
t600 = t594.*2.889644336e+1;
t601 = t593.*2.889644336e+1;
t602 = t593.*1.087689656e+1;
t605 = t596.*2.889644336e+1;
t606 = t597.*2.889644336e+1;
t607 = t596.*1.087689656e+1;
t608 = t594.*6.678442840618982e+2;
t609 = t593.*6.678442840618982e+2;
t612 = t593.*6.185536839278779e+1;
t613 = t594.*1.688943762888624e+2;
t614 = t593.*1.356524863046341e+2;
t616 = t593.*1.870703729528352e-1;
t618 = t596.*6.678442840618982e+2;
t619 = t597.*6.678442840618982e+2;
t620 = t596.*1.356524863046341e+2;
t621 = t597.*1.688943762888624e+2;
t623 = t596.*6.185536839278779e+1;
t624 = t596.*1.870703729528352e-1;
t627 = t4.*t626;
t628 = t8.*t626;
t637 = t36.*t626;
t638 = t39.*t626;
t640 = t42.*t626;
t641 = t45.*t626;
t645 = t516.*t549;
t649 = t75+t292+t597;
t650 = t81+t291+t596;
t651 = t74+t293+t596;
t687 = t516.*t658;
t689 = t3.*t688;
t690 = t7.*t688;
t691 = t431+t529+t598;
t707 = t431+t529+t626;
t728 = -t727;
t733 = t469+t536+t680;
t750 = t516.*t732;
t753 = -t731.*(t348+t5.*(t240-t350));
t787 = t449+t460+t513+t567+t693;
t522 = -t519;
t555 = -t552;
t584 = -t582;
t585 = -t583;
t603 = -t601;
t604 = -t602;
t610 = -t608;
t611 = -t609;
t615 = -t612;
t617 = -t616;
t622 = -t619;
t629 = -t628;
t632 = t628.*7.26735103;
t634 = t627.*1.087689656e+1;
t635 = t628.*1.087689656e+1;
t639 = t628.*(-7.263507131821755e+1);
t642 = t628.*(-6.185536839278779e+1);
t643 = t628.*7.051076542399408e-1;
t644 = t627.*7.051076542399408e-1;
t646 = t441.*t588;
t652 = t4.*t649;
t653 = t8.*t649;
t654 = t5.*t650;
t655 = t9.*t650;
t666 = t38.*t650;
t668 = t37.*t650;
t676 = t526.*t588;
t683 = t153+t315+t319+t606;
t684 = t152+t329+t331+t605;
t692 = -t689;
t695 = t689.*2.889644336e+1;
t696 = t690.*2.889644336e+1;
t697 = t689.*1.087689656e+1;
t699 = t689.*6.678442840618982e+2;
t700 = t690.*6.678442840618982e+2;
t701 = t689.*1.356524863046341e+2;
t702 = t690.*1.688943762888624e+2;
t704 = t689.*6.185536839278779e+1;
t706 = t689.*1.870703729528352e-1;
t708 = t4.*t707;
t709 = t8.*t707;
t716 = t39.*t707;
t717 = t36.*t707;
t720 = t45.*t707;
t721 = t42.*t707;
t734 = t467+t542+t681;
t749 = t162+t330+t333+t336+t446+t448+t607;
t752 = t588.*t730;
t754 = t75+t282+t594+t690;
t759 = -t5.*(t81-t289-t593+t689);
t760 = -t9.*(t81-t289-t593+t689);
t761 = t9.*(t81-t289-t593+t689);
t766 = t5.*(t81-t289-t593+t689).*(-7.26735103);
t768 = t5.*(t81-t289-t593+t689).*7.26735103;
t775 = t5.*(t81-t289-t593+t689).*(-1.336375981993753e+2);
t777 = t38.*(t81-t289-t593+t689);
t778 = t37.*(t81-t289-t593+t689);
t779 = t5.*(t81-t289-t593+t689).*(-1.40259874879e-5);
t781 = t5.*(t81-t289-t593+t689).*1.40259874879e-5;
t782 = t466+t539+t729;
t783 = t248+t258+t386+t409+t413+t621+t624;
t788 = t450+t452+t510+t569+t694;
t789 = t245+t263+t270+t352+t354+t387+t401+t404+t461+t618+1.593951290590465e+3;
t793 = t19.*t28.*t787.*9.543032792050485e-17;
t796 = t504+t507+t558+t561+t685;
t633 = -t632;
t636 = -t635;
t659 = t652.*7.26735103;
t660 = t654.*7.26735103;
t661 = t655.*7.26735103;
t662 = t652.*1.087689656e+1;
t663 = t653.*1.087689656e+1;
t664 = t652.*7.263507131821755e+1;
t665 = t652.*1.336375981993753e+2;
t669 = t653.*1.356524863046341e+2;
t670 = t652.*6.185536839278779e+1;
t671 = t652.*7.051076542399408e-1;
t672 = t653.*7.051076542399408e-1;
t674 = t654.*1.40259874879e-5;
t675 = t655.*1.40259874879e-5;
t678 = -t676;
t703 = -t700;
t705 = -t701;
t710 = -t709;
t711 = t709.*7.26735103;
t713 = t708.*1.087689656e+1;
t714 = t709.*1.087689656e+1;
t718 = t709.*(-1.336375981993753e+2);
t719 = t709.*(-7.263507131821755e+1);
t722 = t709.*(-6.185536839278779e+1);
t723 = t708.*7.051076542399408e-1;
t724 = t709.*7.051076542399408e-1;
t735 = t411+t627+t653;
t736 = t410+t629+t652;
t755 = t4.*t754;
t756 = t8.*t754;
t757 = t78+t283+t593+t692;
t758 = t88+t289+t593+t692;
t765 = t761.*(-7.26735103);
t767 = t761.*7.26735103;
t776 = t761.*(-7.263507131821755e+1);
t780 = t761.*(-1.40259874879e-5);
t784 = t153+t315+t316+t600+t696;
t785 = t152+t325+t331+t603+t695;
t786 = t19.*t28.*t783.*9.543032792050485e-17;
t790 = t253+t266+t275+t356+t359+t373+t403+t423+t462+t622+1.765488401398446;
t794 = t19.*t28.*t788.*5.673626844500105e-17;
t797 = t27.*t796;
t798 = t344.*t789;
t803 = t162+t332+t333+t336+t446+t448+t604+t697;
t826 = t245+t263+t270+t352+t354+t387+t401+t405+t461+t503+t559+t611+t699+1.593951290590465e+3;
t831 = t248+t258+t385+t400+t413+t613+t617+t702+t706;
t667 = -t665;
t673 = -t671;
t712 = -t711;
t715 = -t714;
t725 = -t724;
t737 = t5.*t735;
t738 = t9.*t735;
t751 = t35+t242+t736;
t762 = t755.*7.26735103;
t763 = t755.*1.087689656e+1;
t764 = t756.*1.087689656e+1;
t769 = t755.*1.336375981993753e+2;
t770 = t755.*7.263507131821755e+1;
t771 = t755.*6.185536839278779e+1;
t772 = t756.*1.356524863046341e+2;
t773 = t755.*7.051076542399408e-1;
t774 = t756.*7.051076542399408e-1;
t791 = t159+t322+t342+t445+t451+t634+t663;
t792 = t157+t334+t341+t443+t458+t636+t662;
t795 = -t794;
t799 = t340.*t790;
t804 = t73+t286+t435+t436+t437+t544+t546+t633+t659;
t805 = t411+t708+t756;
t806 = t410+t710+t755;
t822 = t254+t264+t379+t383+t390+t412+t479+t482+t497+t623+t644+t672;
t827 = t253+t266+t275+t356+t359+t373+t403+t420+t462+t505+t566+t610+t703+1.765488401398446;
t829 = (t240-t350).*(t257+t260+t374+t384+t389+t414-t478+t481+t499-t620-t643+t671);
t830 = t344.*t826;
t834 = t19.*t28.*t831.*9.543032792050485e-17;
t836 = t251+t380+t388+t391+t472+t474+t490+t492+t640+t642+t669+t670;
t739 = -t738;
t740 = t737.*7.26735103;
t741 = t738.*7.26735103;
t743 = t737.*7.263507131821755e+1;
t744 = t738.*1.336375981993753e+2;
t746 = t737.*1.40259874879e-5;
t747 = t738.*1.40259874879e-5;
t800 = -t799;
t801 = t521+t655+t737;
t807 = t5.*t805;
t808 = t9.*t805;
t819 = t35+t242+t806;
t823 = t255+t262+t378+t382+t393+t416+t478+t485+t498+t620+t643+t673;
t824 = t159+t322+t342+t445+t451+t713+t764;
t825 = t157+t334+t341+t443+t458+t715+t763;
t828 = t516.*t822;
t832 = t340.*t827;
t835 = t73+t286+t435+t436+t437+t544+t546+t712+t762;
t837 = t340.*t836;
t844 = t254+t264+t375+t383+t390+t412+t479+t482+t497+t615+t704+t723+t774;
t845 = t257+t260+t371+t384+t389+t414+t481+t483+t499+t614+t705+t725+t773;
t855 = t251+t380+t388+t391+t472+t474+t490+t492+t721+t722+t771+t772;
t742 = -t741;
t745 = -t744;
t748 = -t747;
t802 = t519+t654+t739;
t809 = t807.*7.26735103;
t810 = t808.*7.26735103;
t812 = t808.*1.336375981993753e+2;
t813 = t807.*7.263507131821755e+1;
t815 = t807.*1.40259874879e-5;
t816 = t808.*1.40259874879e-5;
t821 = t327+t440+t459+t532+t554+t661+t740;
t833 = -t832;
t838 = t522+t759+t808;
t839 = t521+t761+t807;
t843 = t161+t318+t395+t476+t480+t494+t511+t552+t562+t577+t638+t667+t675+t746;
t846 = t516.*t844;
t847 = -t845.*(t240-t350);
t848 = t845.*(t240-t350);
t849 = -t588.*(t156+t314+t402+t470+t477+t496+t508+t555+t565+t575-t628.*1.336375981993753e+2+t665-t675-t746);
t851 = t588.*(t156+t314+t402+t470+t477+t496+t508+t555+t565+t575-t628.*1.336375981993753e+2+t665-t675-t746);
t856 = t340.*t855;
t811 = -t810;
t814 = -t812;
t817 = -t815;
t818 = -t816;
t820 = t313+t444+t457+t531+t556+t660+t742;
t841 = t327+t440+t459+t532+t554+t767+t809;
t842 = t151+t328+t407+t471+t475+t493+t509+t551+t563+t576+t639+t664+t674+t748;
t853 = t377+t484+t488+t495+t540+t543+t572+t573+t666+t668+t743+t745;
t840 = t313+t444+t457+t531+t556+t768+t811;
t850 = -t842.*(t348+t5.*(t240-t350));
t852 = t842.*(t348+t5.*(t240-t350));
t854 = t516.*t853;
t857 = t156+t314+t402+t470+t477+t496+t508+t555+t565+t575+t718+t769+t780+t817;
t858 = t151+t328+t407+t471+t475+t493+t509+t551+t563+t576+t719+t770+t781+t818;
t862 = t377+t484+t488+t495+t540+t543+t572+t573+t777+t778+t813+t814;
t859 = t588.*t857;
t860 = -t858.*(t348+t5.*(t240-t350));
t861 = t858.*(t348+t5.*(t240-t350));
t863 = t516.*t862;
et1 = t698+t726+t728+t786+t798+t800+t828+t829+t837+t851+t852+t854+t595.*t680+t598.*t681+t649.*t683+t651.*t684+t626.*t729+t650.*t749+t735.*t791+t736.*t792+t751.*t804+t801.*t821+t802.*t820;
et2 = t28.^2.*8.400913676692644e+3;
et3 = 1.896531265228407e+4;
et4 = t305+t426+t427-t434+t502+t581+t590-t591-t682+t686+t687+t750-t752+t731.*(t348+t5.*(t240-t350))+t309.*t626-t300.*t649+t301.*t651+t578.*t650-t533.*t736-t534.*t735-t599.*t751+t630.*t801+t631.*t802;
et5 = 3.03129842504483e-4;
et6 = (dq2.*(et1+et2+et3))./2.0+(dq1.*(t82+t89+t793+t795+t797+t830+t833+t834+t846+t848+t856+t859+t861+t863+t284.*t625+t595.*t733+t598.*t734+t626.*t782+t649.*t784+t651.*t785+t650.*t803+t735.*t824+t736.*t825+t751.*t835+t801.*t841+t802.*t840+1.896531265228407e+4))./2.0+(dq6.*t853)./2.0+(dq3.*(et4+et5))./2.0;
et7 = (dq5.*(t584+t646+t648+t836-t5.*t801.*1.40259874879e-5+t9.*t802.*1.40259874879e-5+t272.*t751))./2.0;
et8 = (dq4.*(t535+t585+t587+t645+t678+t679+t783+t4.*t736.*7.051076542399408e-1+t8.*t735.*7.051076542399408e-1-t209.*t650+t277.*t801+t279.*t802-t751.*(t44-t46)))./2.0;
et9 = t305+t426+t427-t434-t486+t491+t502+t514-t515+t579-t580+t581+t590-t591-t682+t686+t687+t750-t752+t731.*(t348+t5.*(t240-t350))+t631.*(t519-t808+t5.*(t81-t289-t593+t689))+t309.*t707-t300.*t754-t533.*t806-t534.*t805-t599.*t819+t630.*t839+t301.*(t74-t283-t593+t689)+t578.*(t81-t289-t593+t689);
et10 = 3.03129842504483e-4;
et11 = t82+t89+t793+t795+t797+t830+t833+t834+t846+t848+t856+t859+t861+t863+t840.*(t519-t808+t5.*(t81-t289-t593+t689))+t592.*t625+t688.*t733+t691.*t734+t707.*t782+t754.*t784+t805.*t824+t806.*t825+t819.*t835+t839.*t841;
et12 = t56.*(t2.*2.143246204038348e+3+t6.*6.595899367493489e+2+3.22231575312482e+2);
et13 = -t60.*(t2.*(-6.595899367493489e+2)+t6.*2.143246204038348e+3+4.573234736449676e+2);
et14 = t785.*(t74-t283-t593+t689)+t803.*(t81-t289-t593+t689)+2.531266629412227e+5;
et15 = (dq2.*(t82+t89+t698+t726+t728+t786+t798+t800+t828+t829+t837+t851+t852+t854+t820.*(t519-t808+t5.*(t81-t289-t593+t689))+t338.*t592+t680.*t688+t681.*t691+t707.*t729+t683.*t754+t791.*t805+t792.*t806+t804.*t819+t821.*t839+t684.*(t74-t283-t593+t689)+t749.*(t81-t289-t593+t689)+1.896531265228407e+4))./2.0+(dq3.*(et9+et10))./2.0;
et16 = (dq4.*(t535+t585+t587+t645+t678+t679+t831+t279.*(t519-t808+t5.*(t81-t289-t593+t689))+t4.*t806.*7.051076542399408e-1+t8.*t805.*7.051076542399408e-1+t277.*t839-t819.*(t44-t46)-t209.*(t81-t289-t593+t689)))./2.0;
et17 = (dq6.*t862)./2.0+(dq1.*(et11+et12+et13+et14))./2.0+(dq5.*(t584+t646+t648+t855+t9.*(t519-t808+t5.*(t81-t289-t593+t689)).*1.40259874879e-5-t5.*t839.*1.40259874879e-5+t272.*t819))./2.0;
et18 = t252+t381+t388+t391+t439+t442+t473+t474+t490+t492+t547+t548-t628.*1.054594745727878e+2+t640+t652.*1.054594745727878e+2+t669;
et19 = t5.*(t156+t314+t402+t470+t477+t496+t508+t555+t565+t575-t628.*1.336375981993753e+2+t665-t675-t746)+t9.*t842;
et20 = t3.*2.5111251540525e+3-t65.*4.358104279093053e+2;
et21 = t67.*8.018255891962515e+2+t191+t197+t198+t202+t218+t3.*t4.*5.200342652036798e+3+t5.*t86;
et22 = t9.*t90+t5.*t730-t9.*t731;
et23 = t5.*8.018255891962515e+2+t9.*4.358104279093053e+2+t5.*t441+t9.*t438;
et24 = 2.92140771649329e+3;
et25 = dq6.*t310.*(-1.0./2.0)+(dq2.*(et18+et19))./2.0-(dq3.*(et20+et21+et22))./2.0+(dq4.*(t308+t4.*t5.*4.358104279093053e+2-t4.*t9.*8.018255891962515e+2-t5.*t526+t9.*t525))./2.0+(dq5.*(et23+et24))./2.0;
et26 = (dq1.*(t252+t381+t388+t391+t439+t442+t473+t474+t490+t492+t547+t548-t709.*1.054594745727878e+2+t721+t755.*1.054594745727878e+2+t772+t5.*t857+t9.*t858))./2.0;
et27 = (dq6.*t549)./2.0+(dq5.*(t308-t8.*t310+t4.*t5.*t438-t4.*t9.*t441))./2.0+(dq3.*(t523-t4.*t657+t8.*t658+t8.*t732+t5.*t8.*t631.*6.0+t8.*t9.*t630.*6.0+t4.*t5.*t731+t4.*t9.*t730))./2.0+(dq1.*(t831+t4.*t845+t8.*t844+t8.*t862+t5.*t8.*t840.*6.0+t8.*t9.*t841.*6.0+t4.*t5.*t858-t4.*t9.*t857))./2.0;
et28 = (dq2.*(t783+t8.*t822+t8.*t853+t4.*(t257+t260+t374+t384+t389+t414-t478+t481+t499-t620-t643+t671)-t4.*t9.*(t156+t314+t402+t470+t477+t496+t508+t555+t565+t575-t628.*1.336375981993753e+2+t665-t675-t746)+t5.*t8.*t820.*6.0+t8.*t9.*t821.*6.0+t4.*t5.*t842))./2.0;
et29 = (dq4.*(t4.*t312-t8.*t311+t8.*t549+t5.*t8.*t279.*6.0+t8.*t9.*t277.*6.0+t4.*t5.*t525+t4.*t9.*t526+4.098238731829628e+3))./2.0;
et30 = t523-t7.*t209.*4.931128922368695e+1-t3.*t308.*8.595599785252598e-1-t63.*t311+t64.*t312+t63.*t549+t277.*t365+t279.*t364+t145.*t526-t148.*t525+t140.*(t44-t46);
et31 = t3.*t4.^2.*(-3.476976747206118e+1);
et32 = t3.*t8.^2.*(-3.476976747206118e+1);
et33 = t295+t299+t305+t426+t427+t454+t502+t596.*9.559948463095517e-2;
et34 = t597.*8.631091645042425e+1-t145.*(t156+t314+t402+t470+t477+t496+t508+t555+t565+t575-t628.*1.336375981993753e+2+t665-t675-t746);
et35 = t3.*t683.*(-1.291687373922119e+1)+t7.*t684.*1.291687373922119e+1;
et36 = t7.*t749.*4.931128922368695e+1+t3.*t790.*8.595599785252598e-1+t7.*t789.*8.595599785252598e-1-t3.*t836.*8.595599785252598e-1+t63.*t822+t63.*t853-t140.*t804-t148.*t842+t364.*t820;
et37 = t365.*t821+t64.*(t257+t260+t374+t384+t389+t414-t478+t481+t499-t620-t643+t671);
et38 = t3.*t19.*t28.*6.600205872441553e-13;
et39 = t7.*t19.*t28.*(-8.538800689339779e-16);
et40 = t3.*t4.*t792.*(-4.931128922368695e+1)-t3.*t8.*t791.*4.931128922368695e+1;
et41 = 3.03129842504483e-4;
et42 = t3.*(-1.40466005326373e+3);
et43 = t7.*3.416707876634484;
et44 = t3.*t300.*1.291687373922119e+1+t7.*t301.*1.291687373922119e+1+t7.*t524.*8.595599785252598e-1;
et45 = t3.*t530.*8.595599785252598e-1+t51.*t533+t7.*t578.*4.931128922368695e+1+t3.*t656.*8.595599785252598e-1+t63.*t658-t64.*t657+t140.*t599+t63.*t732+t145.*t730-t148.*t731+t364.*t631+t365.*t630;
et46 = t3.*t8.*t534.*4.931128922368695e+1;
et47 = 1.288118518170248e+3;
et48 = t295+t299+t305+t426+t427+t454-t486+t491+t502+t514-t515+t579-t580-t593.*9.559948463095517e-2;
et49 = t594.*8.631091645042425e+1+t689.*9.559948463095517e-2;
et50 = t690.*8.631091645042425e+1-t3.*t784.*1.291687373922119e+1;
et51 = t7.*t785.*1.291687373922119e+1+t7.*t803.*4.931128922368695e+1+t3.*t827.*8.595599785252598e-1;
et52 = t7.*t826.*8.595599785252598e-1-t3.*t855.*8.595599785252598e-1+t63.*t844+t64.*t845+t63.*t862-t140.*t835-t145.*t857-t148.*t858+t364.*t840+t365.*t841;
et53 = t3.*t19.*t28.*2.397546984890625e-13;
et54 = t7.*t19.*t28.*(-3.88386200657948e-16);
et55 = t3.*t4.*t825.*(-4.931128922368695e+1)-t3.*t8.*t824.*4.931128922368695e+1;
et56 = 3.03129842504483e-4;
et57 = (dq4.*(et30+et31+et32))./2.0-(dq5.*(t656+t5.*t365.*1.40259874879e-5-t9.*t364.*1.40259874879e-5+t63.*t310+t140.*t272+t145.*t441+t148.*t438))./2.0+(dq6.*t732)./2.0+(dq2.*(et33+et34+et35+et36+et37+et38+et39+et40+et41))./2.0;
et58 = (dq3.*(et42+et43+et44+et45+et46+et47))./2.0+(dq1.*(et48+et49+et50+et51+et52+et53+et54+et55+et56))./2.0;
K = dq2.*(et6+et7+et8)+dq1.*(et15+et16+et17)+dq4.*(et27+et28+et29)+dq6.*(dq6.*2.100460478666413e+3-(dq5.*t310)./2.0+(dq4.*t549)./2.0+(dq3.*t732)./2.0+(dq2.*t853)./2.0+(dq1.*t862)./2.0)+dq5.*(et25+et26)+dq3.*(et57+et58);
end
